simulink model "Newstart_POTS"  (R2025b)
settings: Solver=VariableStepAuto  StartTime=0.0  StopTime=300  RelTol=1e-3
libraries: pil_lib x1
settings Model: Creator=Lakshay Taneja  LastModifiedBy=Lakshay Taneja

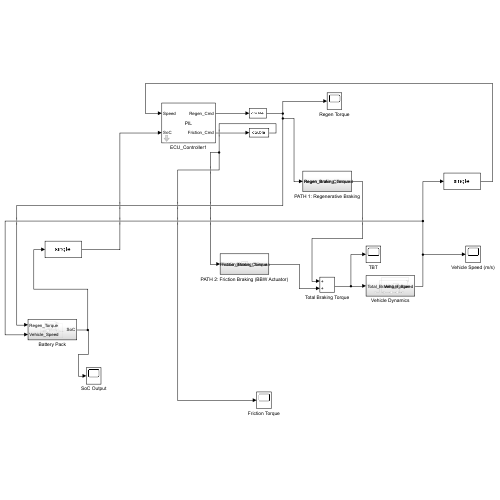
[thumbnail: Simulink's stored preview of the top-level diagram]
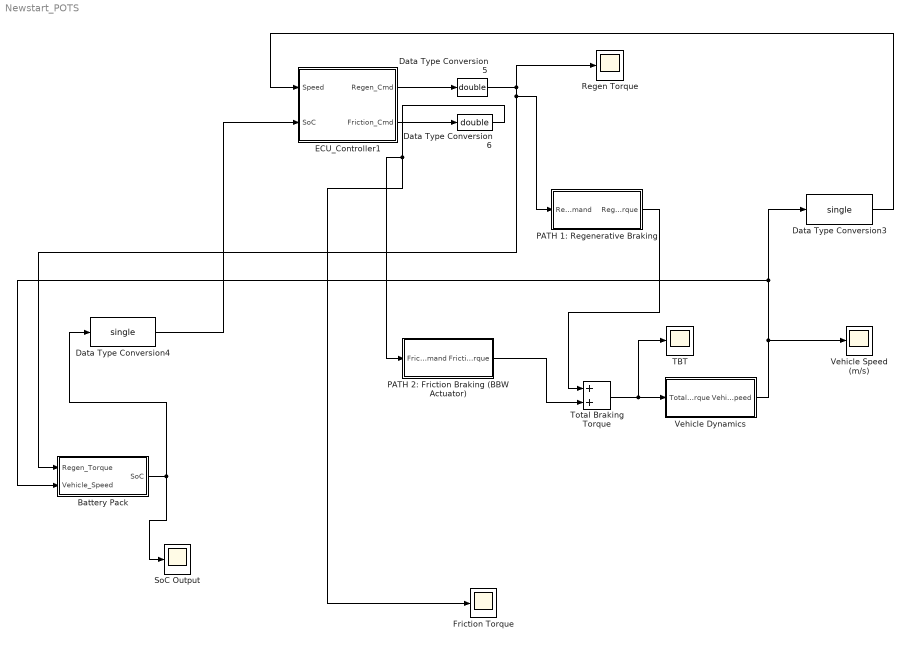
== system Newstart_POTS ==
  Battery Pack : Subsystem
  Data Type Conversion3 : DataTypeConversion  OutDataTypeStr=single  SaturateOnIntegerOverflow=off  RndMeth=Floor
  Data Type Conversion4 : DataTypeConversion  OutDataTypeStr=single  SaturateOnIntegerOverflow=off  RndMeth=Floor
  Data Type Conversion5 : DataTypeConversion  OutDataTypeStr=double  SaturateOnIntegerOverflow=off  RndMeth=Floor
  Data Type Conversion6 : DataTypeConversion  OutDataTypeStr=double  SaturateOnIntegerOverflow=off  RndMeth=Floor
  ECU_Controller1 : Subsystem  DialogController=pil_create_dialog  LoadFcn=|
      | try
      |    if ~strcmp(rtw.pil.getPILVersion, '25.2 (R2025b)_15')
      |       set_param(gcb, 'DialogController', '');
      |       set_param(gcb, 'DialogControllerArgs', '');
      |    end
      | catch e
      |       set_param(gcb, 'DialogController', '');
      |       set_param(gcb, 'DialogControllerArgs', '');
      | end
      mask help: PIL:pil:XILBlockMaskDesc
      mask Display: disp('PIL');
  Friction Torque : Scope
      settings: ActiveDisplayYMinimum=-5400  ActiveDisplayYMaximum=599.99999999999989  DataLoggingVariableName=ScopeData3
  PATH 1: Regenerative Braking : Subsystem
  PATH 2: Friction Braking (BBW Actuator) : Subsystem
  Regen Torque : Scope
      settings: ActiveDisplayYMinimum=-3162.5  ActiveDisplayYMaximum=3462.5  DataLoggingVariableName=ScopeData2
  SoC Output : Scope
      settings: ActiveDisplayYMinimum=0.75712802444298977  ActiveDisplayYMaximum=0.80476355283966783  DataLoggingVariableName=ScopeData4
  TBT : Scope
      settings: ActiveDisplayYMinimum=-1  ActiveDisplayYMaximum=1
  Total Braking Torque : Sum
  Vehicle Dynamics : Subsystem
  Vehicle Speed (m/s) : Scope
      settings: ActiveDisplayYMinimum=-5.3653437153824131  ActiveDisplayYMaximum=48.288093438441727
  wires:
  Total Braking Torque/1 -> TBT/1, Vehicle Dynamics/1(Total_Braking_Torque)
  PATH 2: Friction Braking (BBW Actuator)/1(Friction_Braking_Torque) -> Total Braking Torque/2
  Battery Pack/1(SoC) -> Data Type Conversion4/1, SoC Output/1
  Vehicle Dynamics/1(Vehicle_Speed) -> Battery Pack/2(Vehicle_Speed), Data Type Conversion3/1, Vehicle Speed (m/s)/1
  PATH 1: Regenerative Braking/1(Regen_Braking_Torque) -> Total Braking Torque/1
  Data Type Conversion3/1 -> ECU_Controller1/1(Speed)
  Data Type Conversion4/1 -> ECU_Controller1/2(SoC)
  Data Type Conversion5/1 -> Battery Pack/1(Regen_Torque), PATH 1: Regenerative Braking/1(Regen_Brake_Command), Regen Torque/1
  Data Type Conversion6/1 -> Friction Torque/1, PATH 2: Friction Braking (BBW Actuator)/1(Friction_Brake_Command)
  ECU_Controller1/1(Regen_Cmd) -> Data Type Conversion5/1
  ECU_Controller1/2(Friction_Cmd) -> Data Type Conversion6/1

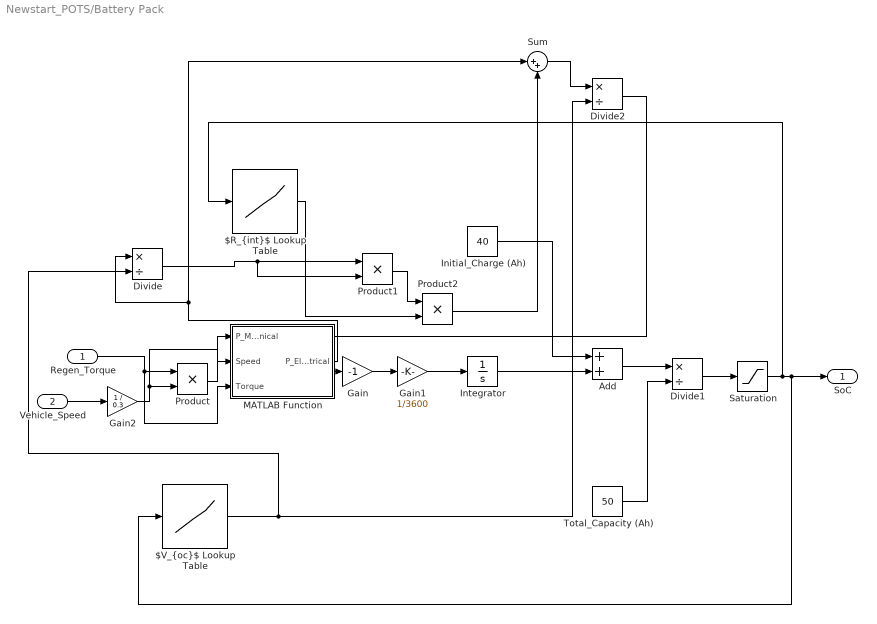
== system Newstart_POTS/Battery Pack ==
  Regen_Torque : Inport
  Vehicle_Speed : Inport  Port=2
  "$R_{int}$ Lookup Table" : Lookup_n-D  NumberOfTableDimensions=1  BreakpointsForDimension1=[0, 0.2, 0.8, 1]  Table=[0.05, 0.02, 0.02, 0.05]  InternalRulePriority=Speed  RndMeth=Simplest
  "$V_{oc}$ Lookup Table" : Lookup_n-D  NumberOfTableDimensions=1  BreakpointsForDimension1=[0, 0.2, 0.8, 1]  Table=[350, 370, 400, 420]  InternalRulePriority=Speed  RndMeth=Simplest
  Add : Sum
  Divide : Product  Inputs=*/
  Divide1 : Product  Inputs=*/
  Divide2 : Product  Inputs=*/
  Gain : Gain  Gain=-1
  Gain1 : Gain  Gain=1/3600
  Gain2 : Gain  Gain=1 / 0.3
  Initial_Charge (Ah) : Constant  Value=40
  Integrator : Integrator
  MATLAB Function : MATLAB Function  TreatAsAtomicUnit=on
  Product : Product
  Product1 : Product
  Product2 : Product
  Saturation : Saturate  UpperLimit=1  LowerLimit=0
  Sum : Sum  Inputs=|++
  Total_Capacity (Ah) : Constant  Value=50
  SoC : Outport
  wires:
  Vehicle_Speed/1 -> Gain2/1
  Regen_Torque/1 -> MATLAB Function/3(Torque), Product/1
  Gain1/1 -> Integrator/1
  Initial_Charge (Ah)/1 -> Add/1
  Integrator/1 -> Add/2
  Add/1 -> Divide1/1
  Total_Capacity (Ah)/1 -> Divide1/2
  Saturation/1 -> "$R_{int}$ Lookup Table"/1, "$V_{oc}$ Lookup Table"/1, SoC/1
  Divide1/1 -> Saturation/1
  Gain/1 -> Gain1/1
  "$V_{oc}$ Lookup Table"/1 -> Divide/2, Divide2/2
  Product1/1 -> Product2/1
  "$R_{int}$ Lookup Table"/1 -> Product2/2
  Product2/1 -> Sum/2
  Sum/1 -> Divide2/1
  Divide2/1 -> Gain/1
  Divide/1 -> Product1/2, Product1/1
  Product/1 -> MATLAB Function/1(P_Mechanical)
  MATLAB Function/1(P_Electrical) -> Sum/1, Divide/1
  Gain2/1 -> MATLAB Function/2(Speed), Product/2

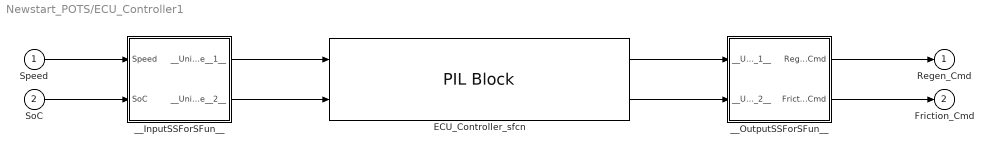
== system Newstart_POTS/ECU_Controller1 ==
  Speed : Inport  OutDataTypeStr=single
  SoC : Inport  Port=2  OutDataTypeStr=single
  ECU_Controller_sfcn : pil_lib/PIL Block  SimulationMode=PIL  IsTopModelPIL=off  CodeDir=ECU_Controller_ert_rtw  AnchorDir=C:\STM32_PIL_POTS  ConfigName=STM32 Targets  XrelIsTopModelCode=on  XrelIsReusable=off  XrelDWorkNames={}  XrelDWorkTypes={}  XrelModelArgVals={}  XrelOrderedParamNames={}  XRelNonFiniteStyle=NONFINITE_UNUSED
  __InputSSForSFun__ : Subsystem
  __OutputSSForSFun__ : Subsystem
  Regen_Cmd : Outport  OutDataTypeStr=single
  Friction_Cmd : Outport  Port=2  OutDataTypeStr=single
  wires:
  Speed/1 -> __InputSSForSFun__/1(Speed)
  SoC/1 -> __InputSSForSFun__/2(SoC)
  __InputSSForSFun__/1(__UniqueOutportName__1__) -> ECU_Controller_sfcn/1
  __InputSSForSFun__/2(__UniqueOutportName__2__) -> ECU_Controller_sfcn/2
  ECU_Controller_sfcn/1 -> __OutputSSForSFun__/1(__UniqueInportName__1__)
  ECU_Controller_sfcn/2 -> __OutputSSForSFun__/2(__UniqueInportName__2__)
  __OutputSSForSFun__/1(Regen_Cmd) -> Regen_Cmd/1
  __OutputSSForSFun__/2(Friction_Cmd) -> Friction_Cmd/1

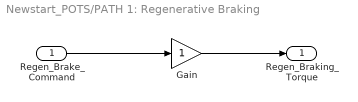
== system Newstart_POTS/PATH 1: Regenerative Braking ==
  Regen_Brake_Command : Inport
  Gain : Gain
  Regen_Braking_Torque : Outport
  wires:
  Regen_Brake_Command/1 -> Gain/1
  Gain/1 -> Regen_Braking_Torque/1

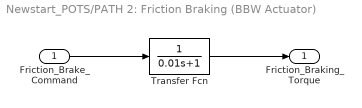
== system Newstart_POTS/PATH 2: Friction Braking (BBW Actuator) ==
  Friction_Brake_Command : Inport
  Transfer Fcn : TransferFcn  Denominator=[0.01 1]
  Friction_Braking_Torque : Outport
  wires:
  Friction_Brake_Command/1 -> Transfer Fcn/1
  Transfer Fcn/1 -> Friction_Braking_Torque/1

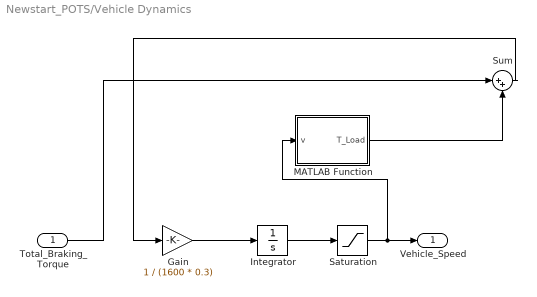
== system Newstart_POTS/Vehicle Dynamics ==
  Total_Braking_Torque : Inport
  Gain : Gain  Gain=1 / (1600 * 0.3)
  Integrator : Integrator
  MATLAB Function : MATLAB Function  TreatAsAtomicUnit=on
  Saturation : Saturate  UpperLimit=inf  LowerLimit=0
  Sum : Sum  Inputs=|++
  Vehicle_Speed : Outport
  wires:
  Total_Braking_Torque/1 -> Sum/1
  Gain/1 -> Integrator/1
  Integrator/1 -> Saturation/1
  Saturation/1 -> MATLAB Function/1(v), Vehicle_Speed/1
  MATLAB Function/1(T_Load) -> Sum/2
  Sum/1 -> Gain/1

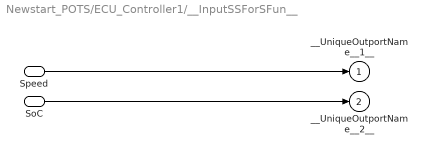
== system Newstart_POTS/ECU_Controller1/__InputSSForSFun__ ==
  Speed : Inport  OutDataTypeStr=single
  SoC : Inport  Port=2  OutDataTypeStr=single
  __UniqueOutportName__1__ : Outport
  __UniqueOutportName__2__ : Outport  Port=2
  wires:
  Speed/1 -> __UniqueOutportName__1__/1
  SoC/1 -> __UniqueOutportName__2__/1

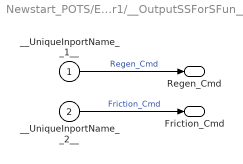
== system Newstart_POTS/ECU_Controller1/__OutputSSForSFun__ ==
  __UniqueInportName__1__ : Inport
  __UniqueInportName__2__ : Inport  Port=2
  Regen_Cmd : Outport  OutDataTypeStr=single
  Friction_Cmd : Outport  Port=2  OutDataTypeStr=single
  wires:
  __UniqueInportName__1__/1 -> Regen_Cmd/1  "Regen_Cmd"
  __UniqueInportName__2__/1 -> Friction_Cmd/1  "Friction_Cmd"

== matlab function Newstart_POTS/Vehicle Dynamics/MATLAB Function ==
  data: v input; T_Load output
function T_Load = Road_Load(v)
    % --- 1. Vehicle Parameters (Synced) ---
    Mass = 1600;       % kg (Synced with your Gain block)
    g = 9.81;          % m/s^2
    rho = 1.225;       % Air density
    Radius = 0.3;      % Wheel Radius (m)
    
    % --- 2. "Sleek EV" Tuning ---
    % We lower these so the air doesn't stop the car too fast.
    % This forces the Regen System to do the work!
    Cd = 0.22;         % Reduced from 0.30 (Sporty Aerodynamics)
    A = 2.2;           % Frontal Area
    Crr = 0.008;       % Reduced from 0.015 (Low Rolling Res Tires)

    % --- 3. Calculate Forces (Newtons) ---
    % Aerodynamic Drag
    F_aero = 0.5 * rho * Cd * A * (v^2);
    
    % Rolling Resistance
    % (tanh makes it smooth at 0 speed to prevent jitter)
    F_roll = Crr * Mass * g * tanh(v * 10); 

    % --- 4. Convert to TORQUE (Nm) ---
    % Critical Fix: Convert Force (N) to Torque (Nm)
    % T = F * r
    % Negative because it opposes motion
    T_Load = -(F_aero + F_roll) * Radius;
end

== matlab function Newstart_POTS/Battery Pack/MATLAB Function ==
  data: P_Mechanical input; P_Electrical output; Speed input; Torque input
function P_Electrical = Motor_Efficiency(P_Mechanical, Speed, Torque)

    % 1. Define Efficiency Map (Simplified)
    % Low efficiency at low speed/torque, High efficiency at rated values.
    % We will use a simple approximation: Base Eff = 0.9, drops at low speeds.
    
    % Avoid divide-by-zero or singular values
    w = abs(Speed) + 1; 
    T = abs(Torque) + 1;
    
    % Simple Efficiency Formula (Empirical)
    % Efficiency improves with speed and torque up to a point
    % Ranges from ~0.6 (at start) to ~0.95 (at cruise)
    Eff_Base = 0.95;
    Loss_Factor = 20; % Higher means more loss at low speeds
    
    Efficiency = Eff_Base - (Loss_Factor / (w * T))^0.5;
    
    % Clamp Efficiency between 0.1 and 0.98 to be safe
    if Efficiency > 0.98
        Efficiency = 0.98;
    elseif Efficiency < 0.1
        Efficiency = 0.1;
    end

    % 2. Apply Efficiency based on Power Flow
    if P_Mechanical >= 0
        % PROPULSION (Battery works harder)
        % P_elec = P_mech / Eff
        P_Electrical = P_Mechanical / Efficiency;
        
    else
        % REGEN (Energy lost to heat)
        % P_elec = P_mech * Eff
        % (Since P_mech is negative, this makes P_elec LESS negative/smaller magnitude)
        P_Electrical = P_Mechanical * Efficiency;
    end
    
end
